simulink model "zad"  (R2013b)
settings: Solver=ode45  StartTime=0.0  StopTime=7  FixedStep=5  RelTol=1e-3
values from neighbouring files (symbols this model uses):
  den = den / den(end)    [optimalModule.m]    (also in pidAlgo.m = input('Please set a denumerator of transfer function: \n'); ziegler.m = conv(den, [1 0]))
  num = num(end)    [model.m]    (also in optimalModule.m = num / den(end); pidAlgo.m = input('Please set a numerator of transfer function: \n'))
  Q0 = q(1)    [pidAlgo.m]    (also in zadanie1.m)
  Q1 = q(2)    [pidAlgo.m]    (also in zadanie1.m)
libraries: simulink x1
settings Model: Creator=Kubo  LastModifiedBy=Kubo

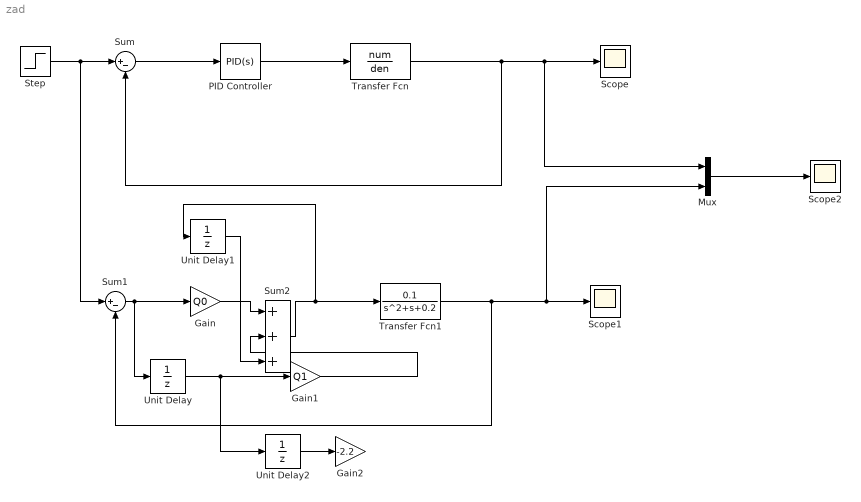
== system zad ==
  Gain : Gain  Gain=Q0
  Gain1 : Gain  Gain=Q1
  Gain2 : Gain  Gain=-2.2
  Mux : Mux  Inputs=2
  PID Controller : simulink/Continuous/PID Controller  Controller=PID  TimeDomain=Continuous-time  SampleTime=1  IntegratorMethod=Forward Euler  FilterMethod=Forward Euler  Form=Parallel  P=19  I=20.25  D=6  N=100  InitialConditionSource=internal  InitialConditionForIntegrator=0  InitialConditionForFilter=0  ExternalReset=none  LimitOutput=off  UpperSaturationLimit=inf  LowerSaturationLimit=-inf  LinearizeAsGain=on  AntiWindupMode=none  Kb=1  TrackingMode=off  Kt=1  PParamMin=[]  PParamMax=[]  IParamMin=[]  IParamMax=[]  DParamMin=[]  DParamMax=[]  NParamMin=[]  NParamMax=[]  KbParamMin=[]  KbParamMax=[]  KtParamMin=[]  KtParamMax=[]  POutMin=[]  POutMax=[]  IOutMin=[]  IOutMax=[]  DOutMin=[]  DOutMax=[]  NOutMin=[]  NOutMax=[]  KbOutMin=[]  KbOutMax=[]  KtOutMin=[]  KtOutMax=[]  IntegratorOutMin=[]  IntegratorOutMax=[]  FilterOutMin=[]  FilterOutMax=[]  SumOutMin=[]  SumOutMax=[]  SumI1OutMin=[]  SumI1OutMax=[]  SumI2OutMin=[]  SumI2OutMax=[]  SumI3OutMin=[]  SumI3OutMax=[]  SumDOutMin=[]  SumDOutMax=[]  SaturationOutMin=[]  SaturationOutMax=[]  IntegratorContinuousStateAttributes=''  IntegratorStateMustResolveToSignalObject=off  IntegratorRTWStateStorageClass=Auto  FilterContinuousStateAttributes=''  FilterStateMustResolveToSignalObject=off  FilterRTWStateStorageClass=Auto
  Scope : Scope
      settings: SaveName=data
  Scope1 : Scope
      settings: SaveName=data1
  Scope2 : Scope
      settings: SaveName=data2
  Step : Step  Time=0  After=6  SampleTime=0
  Sum : Sum  Inputs=|+-
  Sum1 : Sum  Inputs=|+-
  Sum2 : Sum  Inputs=|+++
  Transfer Fcn : TransferFcn  Numerator=num  Denominator=den
  Transfer Fcn1 : TransferFcn  Numerator=0.1  Denominator=[1 1 0.2]
  Unit Delay : UnitDelay  SampleTime=-1
  Unit Delay1 : UnitDelay  SampleTime=-1
  Unit Delay2 : UnitDelay  SampleTime=-1
  wires:
  Step/1 -> Sum1/1, Sum/1
  Sum/1 -> PID Controller/1
  PID Controller/1 -> Transfer Fcn/1
  Transfer Fcn/1 -> Sum/2, Mux/1, Scope/1
  Transfer Fcn1/1 -> Sum1/2, Mux/2, Scope1/1
  Unit Delay/1 -> Unit Delay2/1, Gain1/1
  Gain1/1 -> Sum2/2
  Gain/1 -> Sum2/1
  Sum2/1 -> Unit Delay1/1, Transfer Fcn1/1
  Unit Delay1/1 -> Sum2/3
  Sum1/1 -> Gain/1, Unit Delay/1
  Mux/1 -> Scope2/1
  Unit Delay2/1 -> Gain2/1
